simulink model "quad_6D0F_ASMC"  (R2023a)
settings: Solver=ode1  StartTime=0.0  StopTime=60  FixedStep=0.01  RelTol=1e-3
model workspace (MAT data in the model file):
  omega_n = 20
libraries: sharedtransform x2, matrix_library x1, aerolibutil x1, simulink x1, robotcorelib x1, uavutilslib x1
settings Model: Creator=Adan Daniel  LastModifiedBy=adan

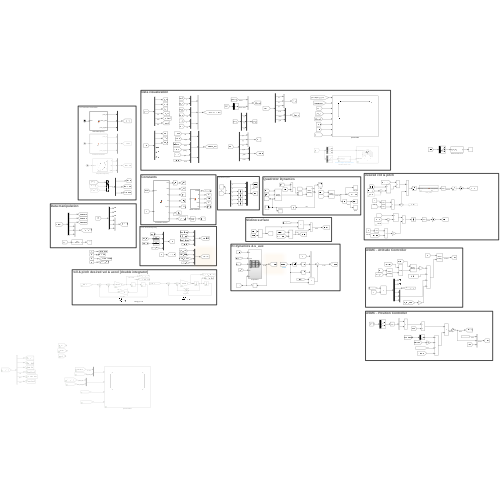
[thumbnail: Simulink's stored preview of the top-level diagram]
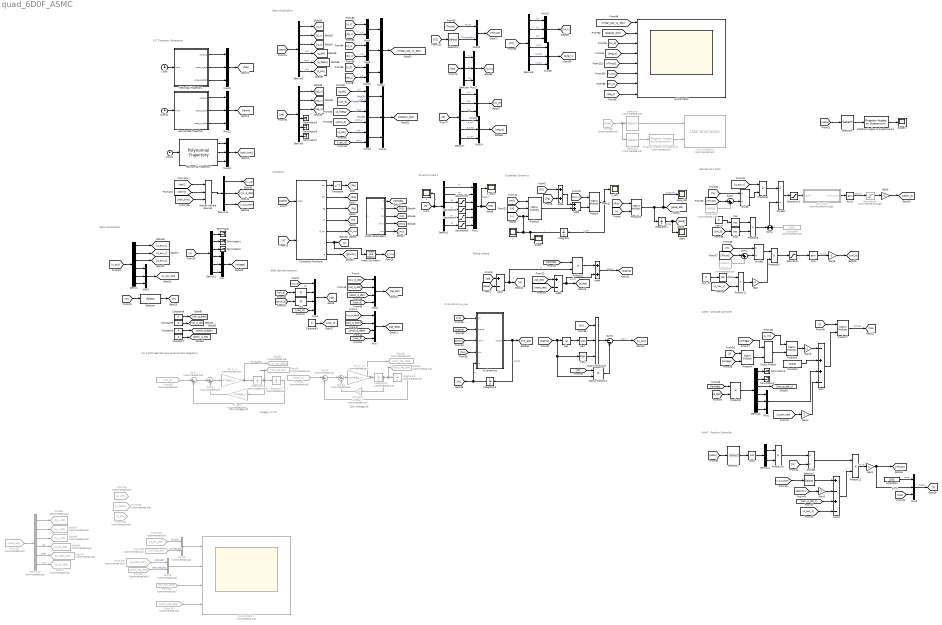
== system quad_6D0F_ASMC ==
  note: omega_n = 20
  note: roll & pitch desired vel & accel [double integrator]
  note: Desired roll & pitch
  note: ASMC - Attitude Controller
  note: Quadrotor Dynamics
  note: XYZ Trajectory Generation
  note: Dynamics Input F
  note: $2\xi \omega_n$
  note: $2\xi \omega_n$
  note: 6DoF desired trajectory
  note: ASMC - Position Controller
  note: Constants
  note: Data manipulation
  note: Data visualization
  note: Sliding surface
  note: Kt dynamics & u_aux
  AMSC parameters : MATLAB Function  TreatAsAtomicUnit=on
  Abs : Abs  SaturateOnIntegerOverflow=off
  Add1 : Sum  Inputs=+-
  Add2 : Sum
  Add3 : Sum  Inputs=+-
  Add4 : Sum
  Add5 : Sum
  Asin : Trigonometry  Operator=asin
  Asin1 : Trigonometry  Operator=asin
  Clock : Clock
  Clock1 : Clock
  Clock2 : Clock
  Constant : Constant  Value=[0;0;0]
  Constant1 : Constant  Commented=on  Value=0.00001
  Constant2 : Constant  Commented=on  Value=0.00001
  Constant{3,5,7..9} (5 alike) : Constant  Value=0
  Constant4 : Constant  Value=[0;0]
  Constant6 : Constant  Commented=on  Value=0.001
  Constants Functions : MATLAB Function  TreatAsAtomicUnit=on
  Cos{,1..3} (4 alike) : Trigonometry  Operator=cos
  Cross Product : matrix_library/Cross Product
  Demux{,1..3,5..8} (8 alike) : Demux  Outputs=6
  Demux10 : Demux  Commented=on  Outputs=6
  Demux11 : Demux  Outputs=3
  Demux4 : Demux  Outputs=2
  Demux9 : Demux  Outputs=3
  Divide : Product  Inputs=*/
  Divide1 : Product  Inputs=*/
  Divide2 : Product  Inputs=*/
  Divide3 : Product  Inputs=/*
  F : Scope
  F_satur : Scope
  From102 : From  Commented=on  GotoTag=roll_hat_ddot
  From103 : From  Commented=on  GotoTag=roll_hat_dot
  From104 : From  Commented=on  GotoTag=q_phi
  From105 : From  Commented=on  GotoTag=q_theta
  From106 : From  Commented=on  GotoTag=q_psi
  From107 : From  Commented=on  GotoTag=pose_dot
  From108 : From  Commented=on  GotoTag=q_phi_dot
  From109 : From  Commented=on  GotoTag=q_theta_dot
  From110 : From  Commented=on  GotoTag=pitch_hat_ddot
  From111 : From  Commented=on  GotoTag=pitch_hat_dot
  From58 : From  Commented=on  GotoTag=pose
  From60 : From  Commented=on  GotoTag=roll_d
  From61 : From  Commented=on  GotoTag=pitch_d
  Gain{,2..3,5..6} (5 alike) : Gain  Gain=-1
  Gain1 : Gain
  Gain4 : Gain
  Goto53 : Goto  Commented=on  GotoTag=roll_hat_ddot
  Goto54 : Goto  Commented=on  GotoTag=roll_hat_dot
  Goto55 : Goto  Commented=on  GotoTag=pitch_hat_ddot
  Goto56 : Goto  Commented=on  GotoTag=pitch_hat_dot
  Goto66 : Goto  Commented=on  GotoTag=q_x_dot
  Goto67 : Goto  Commented=on  GotoTag=q_y_dot
  Goto68 : Goto  Commented=on  GotoTag=q_z_dot
  Goto69 : Goto  Commented=on  GotoTag=q_phi_dot
  Goto70 : Goto  Commented=on  GotoTag=q_theta_dot
  Goto71 : Goto  Commented=on  GotoTag=q_psi_dot
  Helicoidal Trajectory : MATLAB Function  TreatAsAtomicUnit=on
  IC : InitialCondition  Value=0
  IC1 : InitialCondition  Value=0
  Integrator : Integrator  InitialCondition=[0; 0; 0; 0; 0; 0]
  Integrator1 : Integrator  InitialCondition=[2; 0; 0; 0; 0; 0]
  Integrator{2,4..6} (4 alike) : Integrator  Commented=on
  Integrator3 : Integrator  InitialCondition=[0; 0; 0; 0; 0; 0]
  Invert 3x3 Matrix : aerolibutil/Invert  3x3 Matrix
  Kt dynamics : Subsystem
  Lemniscate Trajectory : MATLAB Function  TreatAsAtomicUnit=on
  Manual Variant Source1 : simulink/Signal Routing/Manual Variant Source  NumChoices=3  LabelModeActiveChoice=V_1
  Matrix Multiply3 : Product  Inputs=3
  Matrix Multiply4 : Product
  Mux{,1,3,5,11..17,21..23} (14 alike) : Mux  Inputs=3
  Mux{8..10,20,24..26} (7 alike) : Mux  Inputs=2
  Mux18 : Mux  Commented=on  Inputs=2
  Mux19 : Mux  Commented=on  Inputs=2
  Mux2 : Mux  Inputs=6
  Mux4 : Mux
  Mux6 : Mux
  Mux7 : Mux
  Polynomial Trajectory : robotcorelib/Polynomial Trajectory  WaypointSource=Internal  Waypoints=[0, 0, 0, 0, 0, 0; 0, 0, 0, 0, 0, 0; 0, 2, 5, 2, 5, 2]  TimePoints=[ 0, 12, 24, 36, 48, 60]  TimeInterval=[ 1, 4 ]  Method=Cubic Polynomial  ParameterSource=Internal  VelocityBoundaryCondition=zeros( 3, 6)  AccelerationBoundaryCondition=zeros( 2, 5 )  SimulateUsing=Interpreted execution
  Product{,2,4..5,7} (5 alike) : Product  Multiplication=Matrix(*)
  Product1 : Product  Inputs=3  Multiplication=Matrix(*)
  Product{3,6,8..13} (8 alike) : Product
  QUAD ASMC : Scope  NumInputPorts=8
  QUAD ASMC1 : Scope  Commented=on  NumInputPorts=4
  Rotation Angles to Quaternions : sharedtransform/Rotation Angles to Quaternions  Commented=on  rotationOrder=ZYX  aMode=aMode
  Rotation Angles to Quaternions1 : sharedtransform/Rotation Angles to Quaternions  rotationOrder=ZYX  aMode=aMode
  Saturation : Saturate  UpperLimit=1  LowerLimit=-1
  Saturation1 : Saturate  UpperLimit=1  LowerLimit=-1
  Saturation2 : Saturate  UpperLimit=5.8*4  LowerLimit=0
  Saturation3 : Saturate
  Saturation4 : Saturate
  Saturation5 : Saturate
  Saturation6 : Saturate  Commented=through  UpperLimit=0.1  LowerLimit=-0.1
  Scope : Scope
  Scope1 : Scope
  Selector : Selector  NumberOfDimensions=2  InputPortWidth=3  IndexOptions=Index vector (dialog),Index vector (dialog)  Indices=1,1  OutputSizes=1,1
  Selector1 : Selector  InputPortWidth=3  IndexOptions=Index vector (dialog)  Indices=3  OutputSizes=1
  Selector2 : Selector  InputPortWidth=6  IndexOptions=Index vector (dialog)  Indices=[4 5]  OutputSizes=1
  Selector3 : Selector  InputPortWidth=6  IndexOptions=Index vector (dialog)  Indices=[3]  OutputSizes=1
  Selector4 : Selector  Commented=on  InputPortWidth=6  IndexOptions=Index vector (dialog)  Indices=[1 2 3]  OutputSizes=1
  Selector5 : Selector  Commented=on  InputPortWidth=6  IndexOptions=Index vector (dialog)  Indices=[6 5 4]  OutputSizes=1
  Selector6 : Selector  InputPortWidth=6  IndexOptions=Index vector (dialog)  Indices=[6 5 4]  OutputSizes=1
  Sign1 : Signum
  Sqrt : Sqrt
  Sum : Sum  Inputs=-++-
  Sum1 : Sum  Inputs=|++
  Sum{7..10} (4 alike) : Sum  Commented=on  Inputs=|+-
  Sum2 : Sum  Inputs=|++
  Sum3 : Sum  Inputs=+-+-
  Sum4 : Sum
  Sum6 : Sum  Inputs=|--
  Terminator{,1..7} (8 alike) : Terminator
  Transpose : Math  Operator=transpose
  UAV Animation : uavutilslib/UAV Animation  Commented=on  UAVType=Multirotor  UAVSize=1  InertialZDirection=Up  SampleTime=-1
  asin_satur : MATLAB Function  Commented=through  TreatAsAtomicUnit=on
  pose : Scope
  pose_dot : Scope
  roll_gain : Gain  Commented=on  Gain=omega_n
  roll_gain1 : Gain  Commented=on  Gain=omega_n
  roll_w_n : Gain  Commented=on  Gain=omega_n
  roll_w_n1 : Gain  Commented=on  Gain=omega_n
  v : Scope
  v_dot : Scope
  yaw_d : Constant  Value=0
  yaw_d1 : Constant  Value=0
  wires:
  [v] -> Product2/2
  Product2/1 -> Integrator1/1, pose_dot/1, [pose_dot]  "pose_dot"
  Product/1 -> v_dot/1, Integrator/1  "v_dot"
  Integrator1/1 -> pose/1, [pose]  "pose"
  Integrator/1 -> Scope/1, v/1, [v], Product1/3  "v"
  Add5/1 -> Add2/1
  [M] -> Product1/2
  [Fg] -> Add5/2
  Add2/1 -> Product/2
  [Rib] -> Product2/1
  [Phi] -> Product1/1
  Product1/1 -> Add2/2
  [F2] -> Add5/1
  [M_inv] -> Product/1
  [pose] -> Constants Functions/1(pose)
  [v] -> Constants Functions/2(v)
  Constants Functions/1(Phi) -> Transpose/1
  Constants Functions/4(M) -> [M]
  Constants Functions/3(Fg) -> [Fg]
  Constants Functions/5(M_inv) -> [M_inv]
  Constants Functions/2(Rib) -> [Rib]
  Transpose/1 -> [Phi]
  Clock1/1 -> Polynomial Trajectory/1
  Saturation5/1 -> Mux2/6
  Demux1/5 -> Saturation4/1  "ty"
  Saturation3/1 -> Mux2/4
  Saturation2/1 -> Mux2/3
  Demux1/1 -> Mux2/1  "Fx"
  Demux1/2 -> Mux2/2  "Fy"
  Mux2/1 -> F_satur/1, [F2]  "F_satur"
  [F] -> F/1, Demux1/1  "F"
  Saturation4/1 -> Mux2/5
  Demux1/6 -> Saturation5/1  "tz"
  Demux1/4 -> Saturation3/1  "tx"
  Demux1/3 -> Saturation2/1  "Fz"
  AMSC parameters/5(mu) -> [mu]
  AMSC parameters/2(k1) -> [k1]
  AMSC parameters/3(k2) -> [k2]
  AMSC parameters/4(kmin) -> [kmin]
  [qd] -> Add1/1
  [pose] -> Add1/2
  [qd_dot] -> Add3/1
  AMSC parameters/1(lambda) -> [lambda]
  [lambda] -> Product3/1
  Add1/1 -> Product3/2, [e]  "e"
  Product3/1 -> Add4/1
  Add3/1 -> [e_dot], Add4/2  "e_dot"
  Add4/1 -> [sigma]  "sigma"
  Abs/1 -> Sqrt/1
  Integrator3/1 -> [Kt], Kt dynamics/5(Kt)  "Kt"
  [sigma] -> Matrix Multiply4/2, Sign1/1, Abs/1
  Sign1/1 -> Matrix Multiply3/3
  Matrix Multiply4/1 -> Sum6/2
  [mu] -> Kt dynamics/4(mu)
  Sqrt/1 -> Matrix Multiply3/2
  [k2] -> Matrix Multiply4/1
  [sigma] -> Kt dynamics/2(sigma)
  [k1] -> Kt dynamics/1(K1)
  [Kt] -> Matrix Multiply3/1
  [kmin] -> Kt dynamics/3(Kmin)
  Matrix Multiply3/1 -> Sum6/1
  Kt dynamics/1(Kt_dot) -> Integrator3/1, [Kt_dot]  "Kt_dot"
  Sum6/1 -> [u_aux]  "u_aux"
  [u_aux] -> Demux/1
  Demux/1 -> [u_aux_x]
  Demux/2 -> [u_aux_y]
  Constants Functions/6(J) -> Invert 3x3 Matrix/1, [J]
  [J] -> Product4/1
  [omega] -> Product4/2
  Product4/1 -> Cross Product/2
  [omega] -> Cross Product/1
  Cross Product/1 -> Product5/2
  [J_inv] -> Product5/1
  [lambda] -> Product6/1
  [e_dot] -> Product6/2
  Mux1/1 -> Sum/3
  Demux3/4 -> Mux1/1
  Demux3/6 -> Mux1/3
  Demux3/5 -> Mux1/2
  Product6/1 -> Demux3/1
  Mux3/1 -> [u_aux_tau]
  Demux/4 -> Mux3/1
  Demux/6 -> Mux3/3
  Demux/5 -> Mux3/2
  Product5/1 -> Gain3/1
  Constant/1 -> Sum/2
  [u_aux_tau] -> Gain4/1
  [J] -> Product7/1
  Sum/1 -> Product7/2
  Product7/1 -> [tau]  "torques"
  [M] -> Selector/1
  Selector/1 -> [m]
  [pose_dot] -> Add3/2
  Constant3/1 -> [yaw_d]
  [yaw_d] -> Mux4/4
  [xyz_d] -> Mux4/1
  Mux4/1 -> [qd]
  Demux3/2 -> Terminator4/1
  Demux3/1 -> Terminator3/1
  Demux3/3 -> [lam_e_dot_z]
  Constant4/1 -> Mux5/1  "zeros"
  [tau] -> Mux5/3
  Mux5/1 -> [F]  "forces"
  Demux/3 -> [u_aux_z]
  Divide1/1 -> Saturation1/1
  [u_aux_y] -> Product11/2
  Cos1/1 -> Product9/2
  [m] -> Divide2/1
  Sum1/1 -> Divide/2
  Gain/1 -> Product10/2
  [Thrust] -> Sum2/1
  yaw_d1/1 -> Cos2/1
  Constant1/1 -> Sum1/2
  Product11/1 -> Gain/1
  Cos/1 -> Product9/1
  Product10/1 -> Saturation/1
  Constant2/1 -> Sum2/2
  [roll_d] -> Cos1/1
  Divide2/1 -> Product10/1
  Divide/1 -> Product8/2
  Sum2/1 -> Divide2/2
  [u_aux_x] -> Product8/1
  Cos2/1 -> Product11/1
  Asin1/1 -> Saturation6/1  "pitch_d"
  [Thrust] -> Sum1/1
  Saturation/1 -> Asin/1
  Saturation1/1 -> asin_satur/1(param)
  yaw_d/1 -> Cos/1
  Product8/1 -> Divide1/1
  [m] -> Divide/1
  Asin/1 -> Gain6/1  "roll_d"
  Sum7/1 -> Sum8/1
  From60/1 -> Sum7/1
  Integrator2/1 -> Goto54/1, Integrator4/1, roll_gain/1
  roll_gain/1 -> Sum8/2
  Integrator6/1 -> Sum9/2
  Sum9/1 -> Sum10/1
  Sum8/1 -> roll_w_n/1
  Integrator4/1 -> Sum7/2
  Integrator5/1 -> roll_gain1/1, Goto56/1, Integrator6/1
  roll_w_n/1 -> Integrator2/1, Goto53/1  "roll_d_ddot"
  roll_w_n1/1 -> Goto55/1, Integrator5/1
  roll_gain1/1 -> Sum10/2
  From61/1 -> Sum9/1
  Sum10/1 -> roll_w_n1/1
  [yaw_d] -> Mux6/4
  [roll_d_dot] -> Mux6/2
  [xyz_d_dot] -> Mux6/1
  [pitch_d_dot] -> Mux6/3
  Mux6/1 -> [qd_dot]
  [yaw_d] -> Mux7/4
  [roll_d_ddot] -> Mux7/2
  [xyz_d_ddot] -> Mux7/1
  [pitch_d_ddot] -> Mux7/3
  Mux7/1 -> [qd_ddot]
  [u_aux_z] -> Sum3/4
  [lam_e_dot_z] -> Sum3/3
  [gravity] -> Gain2/1
  Selector1/1 -> Sum3/1
  [xyz_d_ddot] -> Selector1/1
  [pose] -> Selector2/1
  Selector2/1 -> Cos3/1
  Cos3/1 -> Demux4/1
  Demux4/1 -> Product13/1
  Demux4/2 -> Product13/2
  [m] -> Divide3/2
  Sum3/1 -> Product12/2
  Divide3/1 -> Product12/1
  Product13/1 -> Divide3/1
  Product9/1 -> Sum4/1
  Sum4/1 -> Divide1/2
  Constant6/1 -> Sum4/2
  Demux2/1 -> Terminator/1
  Mux/1 -> [omega]
  Demux2/3 -> Terminator2/1
  Demux2/4 -> Mux/1
  Demux2/5 -> Mux/2
  [v] -> Demux2/1
  Demux2/6 -> Mux/3
  Demux2/2 -> Terminator1/1
  Constants Functions/7(g) -> [gravity]
  IC/1 -> Mux4/2
  [roll_d] -> IC/1
  IC1/1 -> Mux4/3
  [pitch_d] -> IC1/1
  Product12/1 -> Gain1/1  "thrust"
  Gain1/1 -> Mux5/2, [Thrust]  "thrust"
  Gain2/1 -> Sum3/2
  Invert 3x3 Matrix/1 -> [J_inv]
  [pose] -> Demux5/1
  Demux5/1 -> [q_x]
  Demux5/2 -> [q_y]
  Demux5/3 -> [q_z]
  Demux5/6 -> [q_psi]  "yaw"
  Demux5/4 -> [q_phi]  "roll"
  Demux5/5 -> [q_theta]  "pitch"
  Demux6/1 -> [qd_x]
  Demux6/2 -> [qd_y]
  [qd] -> Demux6/1
  Demux6/6 -> Terminator7/1
  Demux6/3 -> [qd_z]
  Demux6/5 -> Terminator6/1
  Demux6/4 -> Terminator5/1
  [q_x] -> Mux8/1  "x"
  [qd_x] -> Mux8/2  "x_d"
  [q_y] -> Mux9/1  "y"
  [qd_y] -> Mux9/2  "y_d"
  [q_z] -> Mux10/1  "z"
  [qd_z] -> Mux10/2  "z_d"
  Mux10/1 -> Mux11/3
  Mux9/1 -> Mux11/2
  Mux8/1 -> Mux11/1
  Mux11/1 -> [linear_pos_vs_des]
  [linear_pos_vs_des] -> QUAD ASMC/1
  Mux12/1 -> [angular_pos]
  [e] -> Demux7/1
  Demux7/3 -> Mux13/3  "e_z"
  Demux7/2 -> Mux13/2  "e_y"
  Demux7/1 -> Mux13/1  "e_x"
  Demux7/6 -> Mux14/3  "e_yaw"
  Demux7/4 -> Mux14/1  "e_roll"
  Demux7/5 -> Mux14/2  "e_pitch"
  Mux13/1 -> [lin_e]
  Mux14/1 -> [ang_e]
  Mux15/1 -> [lin_k]
  Demux8/6 -> Mux16/3  "k_yaw"
  [Kt] -> Demux8/1
  Demux8/2 -> Mux15/2  "k_y"
  Demux8/4 -> Mux16/1  "k_roll"
  Demux8/3 -> Mux15/3  "k_z"
  Demux8/1 -> Mux15/1  "k_x"
  Demux8/5 -> Mux16/2  "k_pitch"
  Mux16/1 -> [ang_k]
  [ang_k] -> QUAD ASMC/8
  [angular_pos] -> QUAD ASMC/2
  [lin_e] -> QUAD ASMC/3
  [ang_e] -> QUAD ASMC/4
  [lin_k] -> QUAD ASMC/7
  Constant5/1 -> [pitch_d_ddot]
  Constant7/1 -> [pitch_d_dot]
  Constant9/1 -> [roll_d_dot]
  Constant8/1 -> [roll_d_ddot]
  Saturation6/1 -> Gain5/1
  asin_satur/1(final_param) -> Asin1/1
  Gain3/1 -> Sum/1
  Gain4/1 -> Sum/4
  Gain5/1 -> [pitch_d]
  Gain6/1 -> [roll_d]
  [tau] -> Demux9/1
  Demux9/1 -> Mux17/1  "t_x"
  Demux9/3 -> Mux17/3  "t_z"
  Demux9/2 -> Mux17/2  "t_y"
  Mux17/1 -> [t_xyz]
  [t_xyz] -> QUAD ASMC/6
  Demux10/4 -> Goto69/1  "roll"
  Demux10/5 -> Goto70/1  "pitch"
  Demux10/3 -> Goto68/1
  Demux10/2 -> Goto67/1
  From107/1 -> Demux10/1
  Demux10/6 -> Goto71/1  "yaw"
  Demux10/1 -> Goto66/1
  From108/1 -> Mux18/1  "roll_dot"
  From103/1 -> Mux18/2  "roll_hat_dot"
  Mux18/1 -> QUAD ASMC1/1
  From109/1 -> Mux19/1  "pitch_dot"
  From111/1 -> Mux19/2  "pitch_hat_dot"
  Mux19/1 -> QUAD ASMC1/2
  From102/1 -> QUAD ASMC1/3
  From110/1 -> QUAD ASMC1/4
  [F2] -> Selector3/1
  [Thrust] -> Mux20/1  "Thrust"
  Selector3/1 -> Mux20/2  "Thrust_satur"
  Mux20/1 -> [rThrust]
  [rThrust] -> QUAD ASMC/5
  Mux22/1 -> [lemni]
  Clock/1 -> Helicoidal Trajectory/1(time)
  Lemniscate Trajectory/3(pose_d_ddot) -> Mux22/3
  Helicoidal Trajectory/3(pose_d_ddot) -> Mux21/3
  Clock2/1 -> Lemniscate Trajectory/1(time)
  Lemniscate Trajectory/2(pose_d_dot) -> Mux22/2
  Helicoidal Trajectory/1(pose_d) -> Mux21/1
  Lemniscate Trajectory/1(pose_d) -> Mux22/1
  Helicoidal Trajectory/2(pose_d_dot) -> Mux21/2
  Mux21/1 -> [heli]
  Demux11/1 -> [xyz_d]
  Demux11/3 -> [xyz_d_ddot]
  Demux11/2 -> [xyz_d_dot]
  Manual Variant Source1/1 -> Demux11/1
  Polynomial Trajectory/1 -> Mux23/1
  Polynomial Trajectory/3 -> Mux23/3
  Polynomial Trajectory/2 -> Mux23/2
  Mux23/1 -> [poly_tray]
  [heli] -> Manual Variant Source1/1
  [poly_tray] -> Manual Variant Source1/3
  [lemni] -> Manual Variant Source1/2
  [q_phi] -> Mux24/1  "roll"
  [roll_d] -> Mux24/2  "roll_d"
  [pitch_d] -> Mux25/2  "pitch_d"
  [q_theta] -> Mux25/1  "pitch"
  Mux24/1 -> Mux12/1
  Mux25/1 -> Mux12/2
  [q_psi] -> Mux26/1  "yaw"
  [yaw_d] -> Mux26/2  "yaw_d"
  Mux26/1 -> Mux12/3
  From58/1 -> Selector5/1, Selector4/1
  Selector4/1 -> UAV Animation/1
  Rotation Angles to Quaternions/1 -> UAV Animation/2
  Selector5/1 -> Rotation Angles to Quaternions/1
  [pose] -> Selector6/1
  Selector6/1 -> Rotation Angles to Quaternions1/1
  Rotation Angles to Quaternions1/1 -> Scope1/1

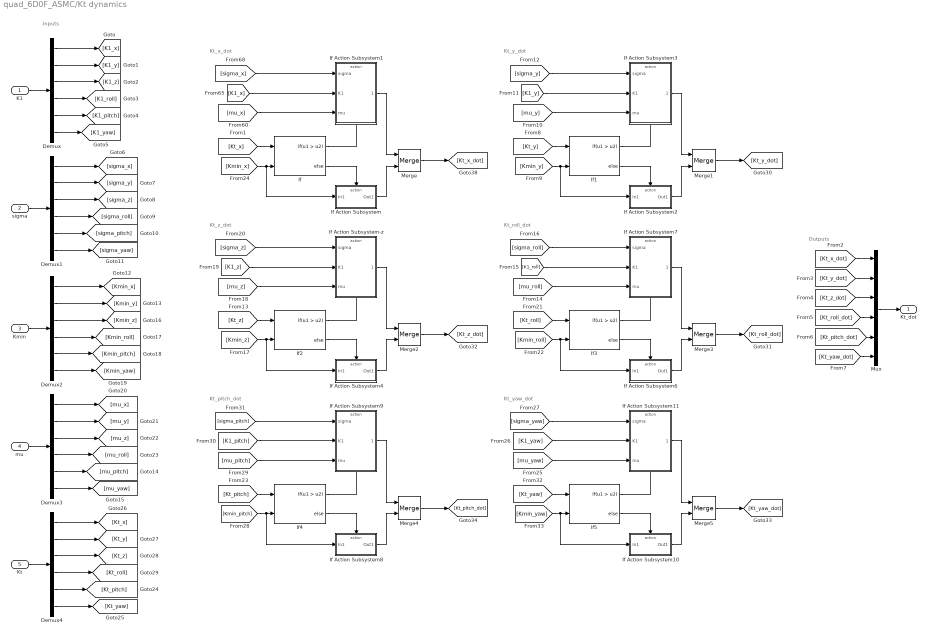
== system quad_6D0F_ASMC/Kt dynamics ==
  note: Outputs
  note: Inputs
  note: Kt_x_dot
  note: Kt_y_dot
  note: Kt_z_dot
  note: Kt_roll_dot
  note: Kt_pitch_dot
  note: Kt_yaw_dot
  K1 : Inport
  sigma : Inport  Port=2
  Kmin : Inport  Port=3
  mu : Inport  Port=4
  Kt : Inport  Port=5
  Demux{,1..4} (5 alike) : Demux  Outputs=6
  If{,1..5} (6 alike) : If  NumInputs=2  IfExpression=u1 > u2
  If Action Subsystem : Subsystem  TreatAsAtomicUnit=on
  If Action Subsystem-z : Subsystem  TreatAsAtomicUnit=on
  If Action Subsystem1 : Subsystem  TreatAsAtomicUnit=on
  If Action Subsystem10 : Subsystem  TreatAsAtomicUnit=on
  If Action Subsystem11 : Subsystem  TreatAsAtomicUnit=on
  If Action Subsystem2 : Subsystem  TreatAsAtomicUnit=on
  If Action Subsystem3 : Subsystem  TreatAsAtomicUnit=on
  If Action Subsystem4 : Subsystem  TreatAsAtomicUnit=on
  If Action Subsystem6 : Subsystem  TreatAsAtomicUnit=on
  If Action Subsystem7 : Subsystem  TreatAsAtomicUnit=on
  If Action Subsystem8 : Subsystem  TreatAsAtomicUnit=on
  If Action Subsystem9 : Subsystem  TreatAsAtomicUnit=on
  Merge{,1..5} (6 alike) : Merge
  Mux : Mux  Inputs=6
  Kt_dot : Outport
  wires:
  [Kt_x] -> If/1
  [sigma_x] -> If Action Subsystem1/1(sigma)
  If/1 -> If Action Subsystem1/Action
  [K1_x] -> If Action Subsystem1/2(K1)
  If Action Subsystem1/1(Kt_x_dot) -> Merge/1
  If Action Subsystem/1(Out1) -> Merge/2
  If/2 -> If Action Subsystem/Action
  Merge/1 -> [Kt_x_dot]
  [Kmin_x] -> If Action Subsystem/1(In1), If/2
  [mu_x] -> If Action Subsystem1/3(mu)
  Merge1/1 -> [Kt_y_dot]
  If1/2 -> If Action Subsystem2/Action
  If Action Subsystem2/1(Out1) -> Merge1/2
  If Action Subsystem3/1(Kt_x_dot) -> Merge1/1
  [Kt_y] -> If1/1
  [K1_y] -> If Action Subsystem3/2(K1)
  [mu_y] -> If Action Subsystem3/3(mu)
  [Kmin_y] -> If Action Subsystem2/1(In1), If1/2
  [sigma_y] -> If Action Subsystem3/1(sigma)
  Merge2/1 -> [Kt_z_dot]
  If Action Subsystem-z/1(Kt_z_dot) -> Merge2/1
  [sigma_z] -> If Action Subsystem-z/1(sigma)
  [Kt_z] -> If2/1
  [mu_z] -> If Action Subsystem-z/3(mu)
  [Kmin_z] -> If Action Subsystem4/1(In1), If2/2
  If3/2 -> If Action Subsystem6/Action
  If Action Subsystem7/1(Kt_x_dot) -> Merge3/1
  Merge3/1 -> [Kt_roll_dot]
  If3/1 -> If Action Subsystem7/Action
  [Kmin_roll] -> If Action Subsystem6/1(In1), If3/2
  If2/2 -> If Action Subsystem4/Action
  [sigma_roll] -> If Action Subsystem7/1(sigma)
  If2/1 -> If Action Subsystem-z/Action
  [K1_roll] -> If Action Subsystem7/2(K1)
  If Action Subsystem6/1(Out1) -> Merge3/2
  [mu_roll] -> If Action Subsystem7/3(mu)
  If Action Subsystem4/1(Out1) -> Merge2/2
  [Kt_roll] -> If3/1
  [K1_z] -> If Action Subsystem-z/2(K1)
  Merge4/1 -> [Kt_pitch_dot]
  If Action Subsystem9/1(Kt_x_dot) -> Merge4/1
  [sigma_pitch] -> If Action Subsystem9/1(sigma)
  [Kt_pitch] -> If4/1
  [mu_pitch] -> If Action Subsystem9/3(mu)
  [Kmin_pitch] -> If Action Subsystem8/1(In1), If4/2
  If5/2 -> If Action Subsystem10/Action
  If Action Subsystem11/1(Kt_x_dot) -> Merge5/1
  Merge5/1 -> [Kt_yaw_dot]
  If5/1 -> If Action Subsystem11/Action
  [Kmin_yaw] -> If Action Subsystem10/1(In1), If5/2
  If4/2 -> If Action Subsystem8/Action
  [sigma_yaw] -> If Action Subsystem11/1(sigma)
  If4/1 -> If Action Subsystem9/Action
  [K1_yaw] -> If Action Subsystem11/2(K1)
  If Action Subsystem10/1(Out1) -> Merge5/2
  [mu_yaw] -> If Action Subsystem11/3(mu)
  If Action Subsystem8/1(Out1) -> Merge4/2
  [Kt_yaw] -> If5/1
  [K1_pitch] -> If Action Subsystem9/2(K1)
  If1/1 -> If Action Subsystem3/Action
  Demux4/6 -> [Kt_yaw]
  Demux4/1 -> [Kt_x]
  Demux1/5 -> [sigma_pitch]
  Demux1/3 -> [sigma_z]
  Demux1/1 -> [sigma_x]
  Demux1/2 -> [sigma_y]
  Kt/1 -> Demux4/1
  Demux4/4 -> [Kt_roll]
  sigma/1 -> Demux1/1
  Demux3/4 -> [mu_roll]
  Demux2/4 -> [Kmin_roll]
  Demux3/1 -> [mu_x]
  Demux2/3 -> [Kmin_z]
  Demux3/3 -> [mu_z]
  mu/1 -> Demux3/1
  Demux3/6 -> [mu_yaw]
  Demux3/5 -> [mu_pitch]
  Demux2/5 -> [Kmin_pitch]
  Demux3/2 -> [mu_y]
  Demux2/6 -> [Kmin_yaw]
  Demux2/1 -> [Kmin_x]
  Demux2/2 -> [Kmin_y]
  Demux/4 -> [K1_roll]
  Demux1/4 -> [sigma_roll]
  Demux4/5 -> [Kt_pitch]
  Demux4/2 -> [Kt_y]
  Demux4/3 -> [Kt_z]
  Demux/1 -> [K1_x]
  K1/1 -> Demux/1
  Demux/6 -> [K1_yaw]
  Demux/5 -> [K1_pitch]
  Demux1/6 -> [sigma_yaw]
  Demux/2 -> [K1_y]
  Kmin/1 -> Demux2/1
  Demux/3 -> [K1_z]
  Mux/1 -> Kt_dot/1
  [Kt_z_dot] -> Mux/3
  [Kt_yaw_dot] -> Mux/6
  [Kt_pitch_dot] -> Mux/5
  [Kt_x_dot] -> Mux/1
  [Kt_y_dot] -> Mux/2
  [Kt_roll_dot] -> Mux/4

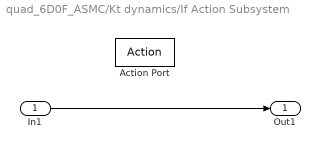
== system quad_6D0F_ASMC/Kt dynamics/If Action Subsystem ==
  In1 : Inport
  Action Port : ActionPort  ActionPortLabel=else
  Out1 : Outport
  wires:
  In1/1 -> Out1/1

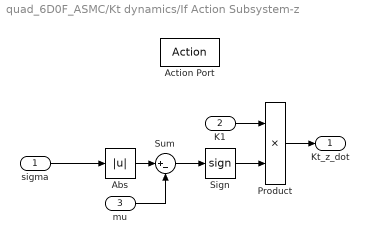
== system quad_6D0F_ASMC/Kt dynamics/If Action Subsystem-z ==
  sigma : Inport
  K1 : Inport  Port=2
  mu : Inport  Port=3
  Action Port : ActionPort  ActionPortLabel=if(u1 > u2)
  Abs : Abs  SaturateOnIntegerOverflow=off
  Product : Product
  Sign : Signum
  Sum : Sum  Inputs=|+-
  Kt_z_dot : Outport
  wires:
  sigma/1 -> Abs/1
  Abs/1 -> Sum/1
  mu/1 -> Sum/2
  Sum/1 -> Sign/1
  Product/1 -> Kt_z_dot/1
  Sign/1 -> Product/2
  K1/1 -> Product/1

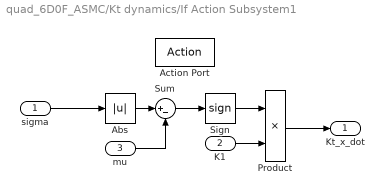
== system quad_6D0F_ASMC/Kt dynamics/If Action Subsystem1 ==
  sigma : Inport
  K1 : Inport  Port=2
  mu : Inport  Port=3
  Action Port : ActionPort  ActionPortLabel=if(u1 > u2)
  Abs : Abs  SaturateOnIntegerOverflow=off
  Product : Product
  Sign : Signum
  Sum : Sum  Inputs=|+-
  Kt_x_dot : Outport
  wires:
  sigma/1 -> Abs/1
  Abs/1 -> Sum/1
  mu/1 -> Sum/2
  Sum/1 -> Sign/1
  Sign/1 -> Product/1
  K1/1 -> Product/2
  Product/1 -> Kt_x_dot/1

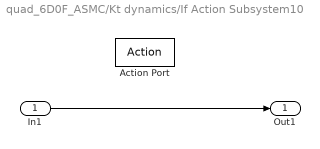
== system quad_6D0F_ASMC/Kt dynamics/If Action Subsystem10 ==
  In1 : Inport
  Action Port : ActionPort  ActionPortLabel=else
  Out1 : Outport
  wires:
  In1/1 -> Out1/1

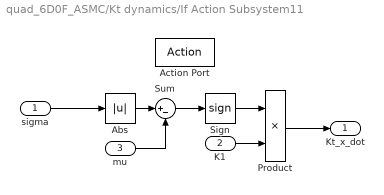
== system quad_6D0F_ASMC/Kt dynamics/If Action Subsystem11 ==
  sigma : Inport
  K1 : Inport  Port=2
  mu : Inport  Port=3
  Action Port : ActionPort  ActionPortLabel=if(u1 > u2)
  Abs : Abs  SaturateOnIntegerOverflow=off
  Product : Product
  Sign : Signum
  Sum : Sum  Inputs=|+-
  Kt_x_dot : Outport
  wires:
  sigma/1 -> Abs/1
  Abs/1 -> Sum/1
  mu/1 -> Sum/2
  Sum/1 -> Sign/1
  Sign/1 -> Product/1
  K1/1 -> Product/2
  Product/1 -> Kt_x_dot/1

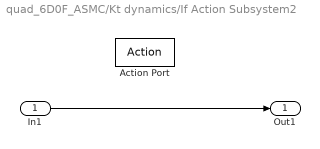
== system quad_6D0F_ASMC/Kt dynamics/If Action Subsystem2 ==
  In1 : Inport
  Action Port : ActionPort  ActionPortLabel=else
  Out1 : Outport
  wires:
  In1/1 -> Out1/1

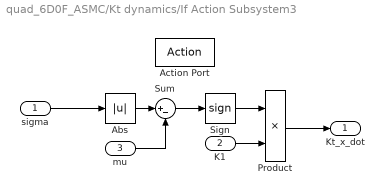
== system quad_6D0F_ASMC/Kt dynamics/If Action Subsystem3 ==
  sigma : Inport
  K1 : Inport  Port=2
  mu : Inport  Port=3
  Action Port : ActionPort  ActionPortLabel=if(u1 > u2)
  Abs : Abs  SaturateOnIntegerOverflow=off
  Product : Product
  Sign : Signum
  Sum : Sum  Inputs=|+-
  Kt_x_dot : Outport
  wires:
  sigma/1 -> Abs/1
  Abs/1 -> Sum/1
  mu/1 -> Sum/2
  Sum/1 -> Sign/1
  Sign/1 -> Product/1
  K1/1 -> Product/2
  Product/1 -> Kt_x_dot/1

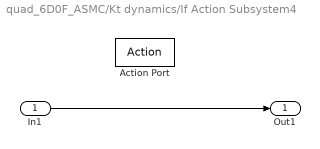
== system quad_6D0F_ASMC/Kt dynamics/If Action Subsystem4 ==
  In1 : Inport
  Action Port : ActionPort  ActionPortLabel=else
  Out1 : Outport
  wires:
  In1/1 -> Out1/1

== system quad_6D0F_ASMC/Kt dynamics/If Action Subsystem6 ==
  In1 : Inport
  Action Port : ActionPort  ActionPortLabel=else
  Out1 : Outport
  wires:
  In1/1 -> Out1/1

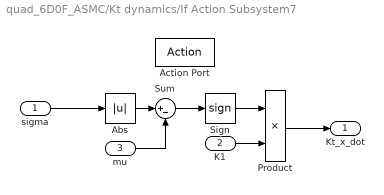
== system quad_6D0F_ASMC/Kt dynamics/If Action Subsystem7 ==
  sigma : Inport
  K1 : Inport  Port=2
  mu : Inport  Port=3
  Action Port : ActionPort  ActionPortLabel=if(u1 > u2)
  Abs : Abs  SaturateOnIntegerOverflow=off
  Product : Product
  Sign : Signum
  Sum : Sum  Inputs=|+-
  Kt_x_dot : Outport
  wires:
  sigma/1 -> Abs/1
  Abs/1 -> Sum/1
  mu/1 -> Sum/2
  Sum/1 -> Sign/1
  Sign/1 -> Product/1
  K1/1 -> Product/2
  Product/1 -> Kt_x_dot/1

== system quad_6D0F_ASMC/Kt dynamics/If Action Subsystem8 ==
  In1 : Inport
  Action Port : ActionPort  ActionPortLabel=else
  Out1 : Outport
  wires:
  In1/1 -> Out1/1

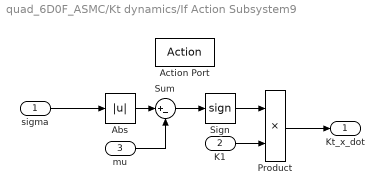
== system quad_6D0F_ASMC/Kt dynamics/If Action Subsystem9 ==
  sigma : Inport
  K1 : Inport  Port=2
  mu : Inport  Port=3
  Action Port : ActionPort  ActionPortLabel=if(u1 > u2)
  Abs : Abs  SaturateOnIntegerOverflow=off
  Product : Product
  Sign : Signum
  Sum : Sum  Inputs=|+-
  Kt_x_dot : Outport
  wires:
  sigma/1 -> Abs/1
  Abs/1 -> Sum/1
  mu/1 -> Sum/2
  Sum/1 -> Sign/1
  Sign/1 -> Product/1
  K1/1 -> Product/2
  Product/1 -> Kt_x_dot/1

== matlab function quad_6D0F_ASMC/AMSC parameters ==
  data: lambda output; unused input; k1 output; k2 output; kmin output; mu output
function [lambda, k1, k2, kmin, mu]= fcn(~)

lambda = [1.25; 1.25; 1.25; 11.25; 11.25; 1];
% bets
k1 = [0.5; 0.5; 2.5; 5; 5; 5];

k2 = [0.75; 0.75; 0.75; 7.5; 7.5; 0.3];

kmin = [0.1; 0.1; 0.1; 0.5; 0.5; 0.1];

mu = [0.01; 0.1; 1; 0.01; 0.01; 0.1];

== matlab function quad_6D0F_ASMC/asin_satur ==
  data: param input; final_param output
function final_param = asin_saturation(param)

if param > 1
    final_param = 1;
elseif param < -1
    final_param = -1;
else
    final_param = param;
end

== matlab function quad_6D0F_ASMC/Constants Functions ==
  data: Phi output; Rib output; Fg output; pose input; M output; M_inv output; v input; J output; g output
function [Phi, Rib, Fg, M, M_inv, J, g]   = fcn(pose, v)

%% System constants
m = 2; %5 mass 2.2 kg
l = 0.25; % m
g = 9.81; % gravity
Jxx =  0.0411; % kg m²
Jyy = 0.0478; % kg m²
Jzz = 0.0599; % kg m²
kT = 3.4e-5;
kQ = 3.4e-6;
%% Phi vector 6d

uu = v(1);
vv = v(2);
ww = v(3);
pp = v(4);
qq = v(5);
rr = v(6);


Phi = [0, -rr, qq, 0, -ww, vv;
        rr, 0, -pp , ww, 0, -uu;
        -qq, pp, 0,  -vv, uu, 0;
        0, 0, 0, 0, -rr, qq; 
        0, 0, 0, rr, 0, -pp;
        0, 0, 0, -qq, pp, 0];
%% Fg and Rib calculation

roll = pose(4);
pitch = pose(5);
yaw = pose(6);


Rib = [cos(yaw)*cos(pitch), -cos(roll)*sin(yaw) + cos(yaw)*sin(roll)*sin(pitch), sin(roll)*sin(yaw) + cos(roll)*cos(yaw)*sin(pitch), 0, 0, 0;
       cos(pitch)*sin(yaw), cos(roll)*cos(yaw) + sin(yaw)*sin(pitch)*sin(roll), -cos(yaw)*sin(roll) + sin(yaw)*sin(pitch)*cos(roll), 0, 0, 0;
       -sin(pitch), cos(pitch)*sin(roll), cos(pitch)*cos(roll), 0, 0, 0;
       0, 0, 0, 1, sin(roll)*tan(pitch), cos(roll)*tan(pitch);
       0, 0, 0, 0, cos(roll), -sin(roll);
       0, 0, 0, 0, sin(roll)/cos(pitch), cos(roll)/cos(pitch)];

Fg = [m*g*sin(pitch);
      -m*g*cos(pitch)*sin(roll);
      -m*g*cos(pitch)*cos(roll);
      0;
      0;
      0];

%% M matrix

M = [m, 0, 0, 0, 0, 0;
    0, m, 0, 0, 0, 0;
    0, 0, m, 0, 0, 0;
    0, 0, 0, Jxx, 0, 0;
    0, 0, 0, 0, Jyy, 0;
    0, 0, 0, 0, 0, Jzz];

M_inv = inv(M);

%% Allocation matrix

% allo = [0, 0, 0, 0, 0, 0;
%         0, 0, 0, 0, 0, 0;
%         kT, kT, kT, kT, kT, kT;
%         -kT*l, kT*l, kT*l/2, -kT*l/2, -kT*l/2, kT*l/2;
%         0, 0, -sqrt(3)*kT*l/2, sqrt(3)*kT*l/2, -sqrt(3)*kT*l/2, sqrt(3)*kT*l/2;
%         kQ, -kQ, kQ, -kQ, -kQ, kQ,];
% 
% allo = pinv(allo);

J = [Jxx, 0, 0;
     0, Jyy, 0;
     0, 0, Jzz];

== matlab function quad_6D0F_ASMC/Helicoidal Trajectory ==
  data: time input; pose_d output; pose_d_dot output; pose_d_ddot output
function [pose_d, pose_d_dot, pose_d_ddot]= fcn(time)

pos_z = time / 12;
f = 0.15;
arg = f * (time - 5);
r = 2;

% hover for 5 s | include inclination in roll
% 5 metros al menos

if (time < 5)
    pos_x = 2;
    pos_y = 0;
    % roll = 0;
else
    pos_x = r * cos (arg);
    pos_y = r * sin (arg);
    % roll = 0.15;
end

% roll = 0;
% yaw = time * 0;

pose_d = [pos_x;
          pos_y;
          pos_z];
          % roll;
          % 0;
          % yaw];

pos_z_dot = 1 / 12;

% hover for 5 s
if (time < 5)
    pos_x_dot = 0;
    pos_y_dot = 0;
else
    pos_x_dot = - f * r * sin(arg);
    pos_y_dot = f * r * cos(arg);
end

% yaw_dot = 0;

pose_d_dot = [pos_x_dot;
              pos_y_dot;
              pos_z_dot];
              % 0;
              % 0;
              % yaw_dot];

pos_z_ddot = 0;
% hover for 5 s
if (time < 5)
    pos_x_ddot = 0;
    pos_y_ddot = 0;
else
    pos_x_ddot = - f * f * r * cos(arg);
    pos_y_ddot = - f * f * r * sin(arg);
end

% yaw_ddot = 0;

pose_d_ddot = [pos_x_ddot;
               pos_y_ddot;
               pos_z_ddot];
               % 0;
               % 0;
               % yaw_ddot];

== matlab function quad_6D0F_ASMC/Lemniscate Trajectory ==
  data: time input; pose_d output; pose_d_dot output; pose_d_ddot output
function [pose_d, pose_d_dot, pose_d_ddot]= fcn(time)

%% Positions

arg = time / 4;

pos_x = cos(arg) ./ (1 + sin(arg) .* sin(arg));
pos_y = cos(arg) .* sin(arg) ./ (1 + sin(arg) .* sin(arg));
pos_z = time / 12;

% yaw = time * 0;

pose_d = [pos_x;
          pos_y;
          pos_z];
          % 0;
          % 0;
          % yaw];

%% Velocities

pos_z_dot = 1 / 12;
pos_x_dot = 0;
pos_y_dot = 0;
% yaw_dot = 0;

pose_d_dot = [pos_x_dot;
              pos_y_dot;
              pos_z_dot];
              % 0;
              % 0;
              % yaw_dot];

%% Accelerations

pos_z_ddot = 0;
pos_x_ddot = 0;
pos_y_ddot = 0;
% yaw_ddot = 0;

pose_d_ddot = [pos_x_ddot;
               pos_y_ddot;
               pos_z_ddot];
               % 0;
               % 0;
               % yaw_ddot];
